simulink model "sixDOF4"  (R2024a)
settings: Solver=VariableStepAuto  StartTime=0.0  StopTime=30  MinStep=0.001  RelTol=1e-3
PreLoadFcn:
  | load("C:\Users\craig\OneDrive\Desktop\Matlab\TVC\Workspaces\rocketProps.mat");
values from neighbouring files (symbols this model uses):
  AoA = [-88.914 -74.145 -55.955 -43.246 -35.663 -31.356 -27.884 -25.044 -22.757 -21.029 -19.522 -18.257 ... (59 elements, 59x1)]    [rocketProps.mat]
  Cn = [-5.771 -4.929 -4.21 -3.639 -3.162 -2.748 -2.412 -2.115 -1.835 -1.564 -1.294 -1.003 ... (59 elements, 59x1)]    [rocketProps.mat]
  thrust = [13 82 98 100 90 86 93 96 96 92 88 83 ... (16 elements, 16x1)]    [rocketProps.mat]
  time = [0.01 0.02 0.03 0.04 0.05 0.06 0.12 0.2 0.3 0.7 0.9 1.07 ... (16 elements, 16x1)]    [rocketProps.mat]
undefined symbols (not defined in the file or in its folder): magnitude
libraries: sharedtransform x2, simulink x2, aerolibanim x1, vrlib x1
settings Model: NumberOfSteps=100  Creator=craig  LastModifiedBy=craig
settings SolverCC: MaxConsecutiveMinStep=2
settings DebuggingCC: UnderSpecifiedDataTypeMsg=warning  UnderSpecifiedDimensionMsg=warning

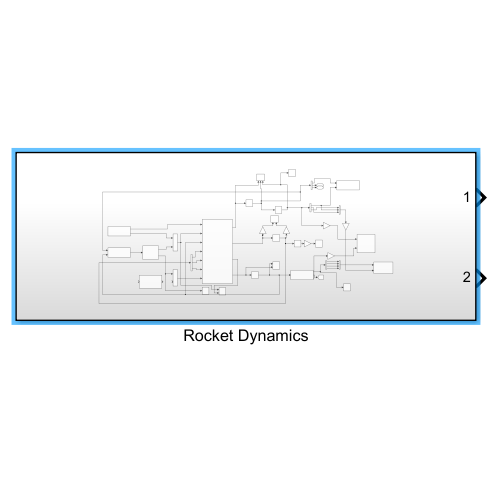
[thumbnail: Simulink's stored preview of the top-level diagram]
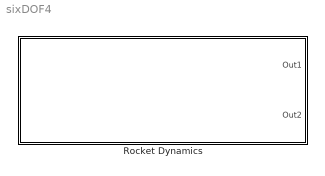
== system sixDOF4 ==
  Rocket Dynamics : Subsystem

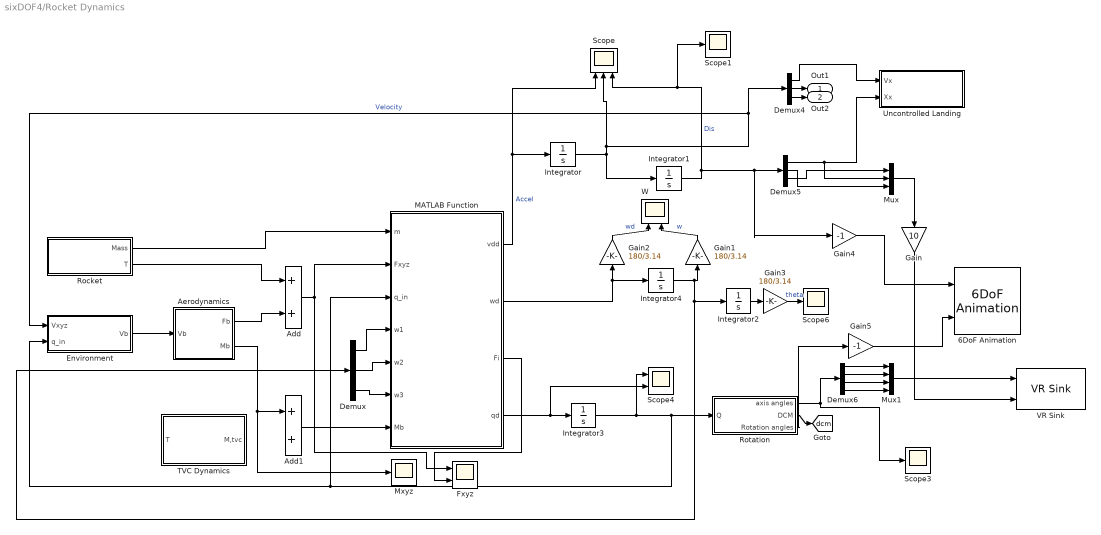
== system sixDOF4/Rocket Dynamics ==
  6DoF Animation : aerolibanim/6DoF Animation  u1=[0 4000 -2000 2000 -5000 -3000]  u2=0.1  u3=100  u4=[4000 0 -5000]  u5=Fixed position  u6=[2000 500 -3150]  u7=10  u8=on
  Add : Sum
  Add1 : Sum
  Aerodynamics : Subsystem
  Demux : Demux  Outputs=3
  Demux4 : Demux  Outputs=3
  Demux5 : Demux  Outputs=3
  Demux6 : Demux
  Environment : Subsystem
  Fxyz : Scope  NumInputPorts=2
  Gain : Gain  Gain=10
  Gain1 : Gain  Gain=180/3.14
  Gain2 : Gain  Gain=180/3.14
  Gain3 : Gain  Gain=180/3.14
  Gain4 : Gain  Gain=-1
  Gain5 : Gain  Gain=-1
  Integrator : Integrator  InitialCondition=[0; 0; 0]
  Integrator1 : Integrator
  Integrator2 : Integrator  InitialCondition=[0; 0; 0]
  Integrator3 : Integrator  InitialCondition=[1; 0; 0; 0]
  Integrator4 : Integrator  InitialCondition=[0; 0; 0]
  MATLAB Function : MATLAB Function  TreatAsAtomicUnit=on
  Mux : Mux  Inputs=3
  Mux1 : Mux
  Mxyz : Scope
  Rocket : Subsystem
  Rotation : Subsystem
  Scope : Scope  NumInputPorts=3
  Scope1 : Scope
  Scope3 : Scope
  Scope4 : Scope  NumInputPorts=2
  Scope6 : Scope
  TVC Dynamics : Subsystem
  Uncontrolled Landing : Subsystem
  VR Sink : vrlib/VR Sink  InstantiateOnLoad=on  SampleTime=0.1  ViewEnable=on  RemoteChange=off  RemoteView=off  FieldsWritten=MyTransform.rotation.4.1.1.double#MyTransform.translation.3.1.1.double  WorldFileName=C:\Users\craig\OneDrive\Desktop\Matlab\TVC\Animations\BestViewpoint.wrl  AutoView=off  VideoDimensions=[]  AllowVariableSize=off
  W : Scope  NumInputPorts=2
  Out1 : Outport
  Out2 : Outport  Port=2
  tag scope: dcm=global
  wires:
  Integrator3/1 -> Scope4/1, Rotation/1(Q), MATLAB Function/3(q_in), Environment/2(q_in)
  Add/1 -> Fxyz/1, MATLAB Function/2(Fxyz)
  Integrator2/1 -> Gain3/1
  Integrator4/1 -> Integrator2/1, Demux/1, Gain1/1
  Integrator/1 -> Integrator1/1, Demux4/1, Environment/1(Vxyz), Scope/2  "Velocity"
  Demux/1 -> MATLAB Function/4(w1)
  Integrator1/1 -> Scope1/1, Scope/3, Gain4/1, Demux5/1  "Dis"
  Demux5/1 -> Uncontrolled Landing/2(Xx), Mux/2
  MATLAB Function/3(Fi) -> Fxyz/2
  Environment/1("Vb ") -> Aerodynamics/1(Vb)
  Gain/1 -> VR Sink/2
  Mux/1 -> Gain/1
  Gain3/1 -> Scope6/1  "theta"
  Demux/3 -> MATLAB Function/6(w3)
  MATLAB Function/1(vdd) -> Integrator/1, Scope/1  "Accel"
  Aerodynamics/2(Mb) -> Add1/1, Mxyz/1
  Demux/2 -> MATLAB Function/5(w2)
  Demux4/3 -> Out2/1
  MATLAB Function/2(wd) -> Integrator4/1, Gain2/1
  MATLAB Function/4(qd) -> Scope4/2, Integrator3/1
  Rotation/1(axis angles) -> Scope3/1, Demux6/1
  Rocket/2(T) -> Add/1
  Gain1/1 -> W/2  "w"
  Rocket/1(Mass) -> MATLAB Function/1(m)
  Aerodynamics/1(Fb) -> Add/2
  Gain2/1 -> W/1  "wd"
  Rotation/2(DCM) -> [dcm]
  Demux4/1 -> Uncontrolled Landing/1(Vx)
  Rotation/3(Rotation angles) -> Gain5/1
  Gain4/1 -> 6DoF Animation/1
  Gain5/1 -> 6DoF Animation/2
  Demux4/2 -> Out1/1
  Add1/1 -> MATLAB Function/7(Mb)
  Mux1/1 -> VR Sink/1
  Demux5/3 -> Mux/1
  Demux5/2 -> Mux/3
  Demux6/2 -> Mux1/2
  Demux6/3 -> Mux1/3
  Demux6/1 -> Mux1/1
  Demux6/4 -> Mux1/4

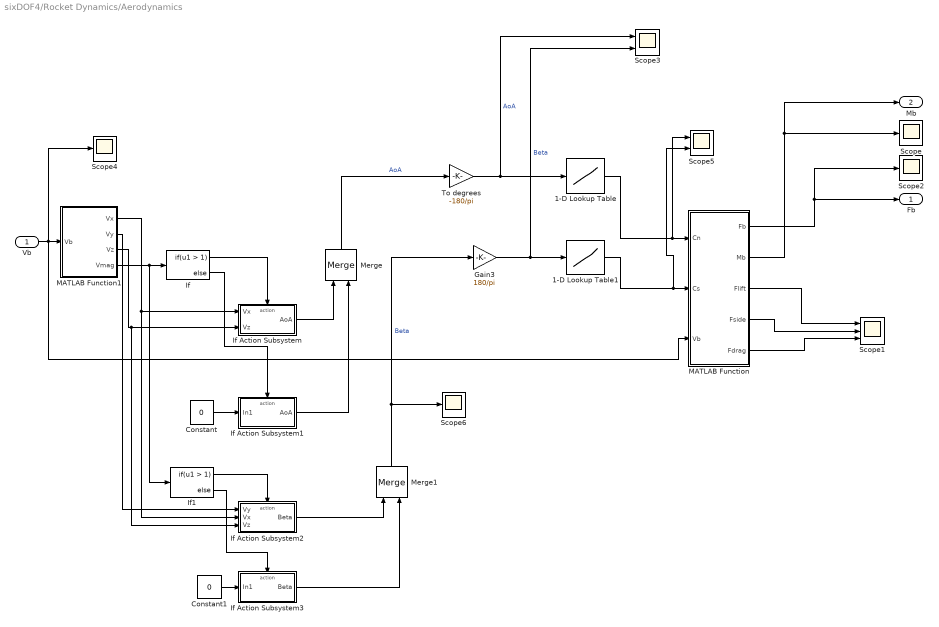
== system sixDOF4/Rocket Dynamics/Aerodynamics ==
  Vb : Inport
  1-D Lookup Table : Lookup_n-D  NumberOfTableDimensions=1  BreakpointsForDimension1=AoA  Table=Cn  InternalRulePriority=Speed  RndMeth=Simplest
  1-D Lookup Table1 : Lookup_n-D  NumberOfTableDimensions=1  BreakpointsForDimension1=AoA  Table=Cn  InternalRulePriority=Speed  RndMeth=Simplest
  Constant : Constant  Value=0
  Constant1 : Constant  Value=0
  Gain3 : Gain  Gain=180/pi
  If : If  IfExpression=u1 > 1
  If Action Subsystem : Subsystem  TreatAsAtomicUnit=on
  If Action Subsystem1 : Subsystem  TreatAsAtomicUnit=on
  If Action Subsystem2 : Subsystem  TreatAsAtomicUnit=on
  If Action Subsystem3 : Subsystem  TreatAsAtomicUnit=on
  If1 : If  IfExpression=u1 > 1
  MATLAB Function : MATLAB Function  TreatAsAtomicUnit=on
  MATLAB Function1 : MATLAB Function  TreatAsAtomicUnit=on
  Merge : Merge
  Merge1 : Merge
  Scope{,2,4,6} (4 alike) : Scope
  Scope1 : Scope  NumInputPorts=3
  Scope3 : Scope  NumInputPorts=2
  Scope5 : Scope  NumInputPorts=2
  To degrees : Gain  Gain=-180/pi
  Fb : Outport
  Mb : Outport  Port=2
  wires:
  MATLAB Function/3(Flift) -> Scope1/1
  MATLAB Function/2(Mb) -> Scope/1, Mb/1
  MATLAB Function/1(Fb) -> Scope2/1, Fb/1
  To degrees/1 -> Scope3/1, 1-D Lookup Table/1  "AoA"
  Gain3/1 -> Scope3/2, 1-D Lookup Table1/1  "Beta"
  MATLAB Function/5(Fdrag) -> Scope1/3
  Vb/1 -> Scope4/1, MATLAB Function/3(Vb), MATLAB Function1/1(Vb)
  If/2 -> If Action Subsystem1/Action
  MATLAB Function1/4(Vmag) -> If1/1, If/1
  Constant/1 -> If Action Subsystem1/1(In1)
  MATLAB Function1/1(Vx) -> If Action Subsystem2/2(Vx), If Action Subsystem/1(Vx)
  MATLAB Function1/3(Vz) -> If Action Subsystem2/3(Vz), If Action Subsystem/2(Vz)
  If/1 -> If Action Subsystem/Action
  If Action Subsystem/1(AoA) -> Merge/1
  If Action Subsystem1/1(AoA) -> Merge/2
  Merge/1 -> To degrees/1  "AoA"
  MATLAB Function1/2(Vy) -> If Action Subsystem2/1(Vy)
  Constant1/1 -> If Action Subsystem3/1(In1)
  If Action Subsystem2/1(Beta) -> Merge1/1
  If Action Subsystem3/1(Beta) -> Merge1/2
  If1/2 -> If Action Subsystem3/Action
  If1/1 -> If Action Subsystem2/Action
  1-D Lookup Table1/1 -> Scope5/2, MATLAB Function/2(Cs)
  1-D Lookup Table/1 -> Scope5/1, MATLAB Function/1(Cn)
  MATLAB Function/4(Fside) -> Scope1/2
  Merge1/1 -> Gain3/1, Scope6/1  "Beta"

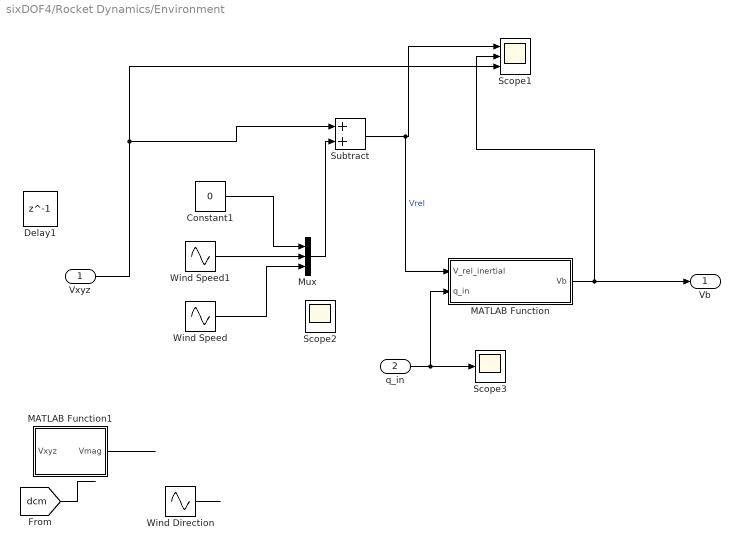
== system sixDOF4/Rocket Dynamics/Environment ==
  Vxyz : Inport
  q_in : Inport  Port=2
  Constant1 : Constant  Value=0
  Delay1 : Delay  DelayLength=1
  MATLAB Function : MATLAB Function  TreatAsAtomicUnit=on
  MATLAB Function1 : MATLAB Function  TreatAsAtomicUnit=on
  Mux : Mux  Inputs=3
  Scope1 : Scope  NumInputPorts=3
  Scope2 : Scope
  Scope3 : Scope
  Subtract : Sum
  Wind Direction : Sin  Amplitude=5  Bias=45  Frequency=2*pi*0.25  SampleTime=0
  Wind Speed : Sin  Amplitude=5  Bias=3.5  Frequency=2*pi*0.25  SampleTime=0
  Wind Speed1 : Sin  Amplitude=5  Bias=3.5  Frequency=2*pi*0.25  SampleTime=0
  "Vb " : Outport
  wires:
  Subtract/1 -> MATLAB Function/1(V_rel_inertial), Scope1/1  "Vrel"
  Vxyz/1 -> Subtract/1, Scope1/3
  [dcm] -> ?
  MATLAB Function1/1(Vmag) -> ?
  MATLAB Function/1(Vb) -> "Vb "/1, Scope1/2
  Wind Direction/1 -> ?
  Constant1/1 -> Mux/1
  q_in/1 -> MATLAB Function/2(q_in), Scope3/1
  Mux/1 -> Subtract/2
  Wind Speed1/1 -> Mux/2
  Wind Speed/1 -> Mux/3

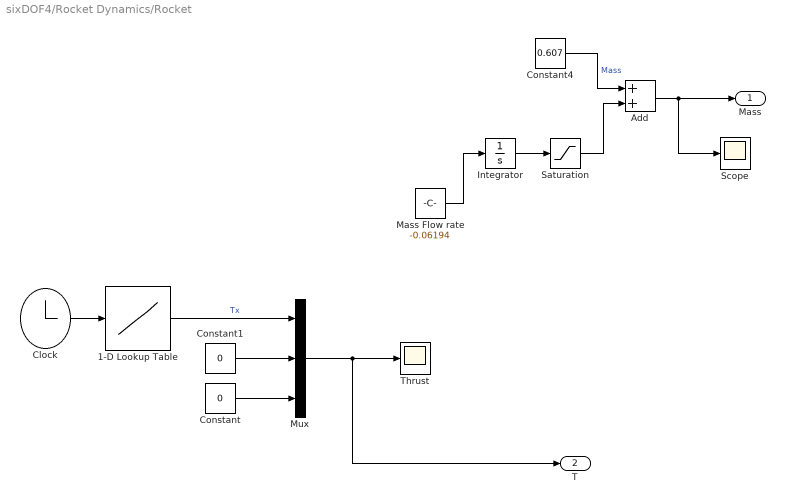
== system sixDOF4/Rocket Dynamics/Rocket ==
  1-D Lookup Table : Lookup_n-D  NumberOfTableDimensions=1  BreakpointsForDimension1=time  Table=thrust  TableMin=[0]  TableDataTypeStr=Inherit: Inherit from 'Table data'  ExtrapMethod=Clip  UseLastTableValue=on  InternalRulePriority=Speed  RndMeth=Simplest
  Add : Sum
  Clock : Clock
      settings: Decimation=100
  Constant : Constant  Value=0
  Constant1 : Constant  Value=0
  Constant4 : Constant  Value=0.607
  Integrator : Integrator  InitialCondition=0.188
  Mass Flow rate : Constant  Value=-0.06194
  Mux : Mux  Inputs=3
  Saturation : Saturate  LowerLimit=0.105
  Scope : Scope
  Thrust : Scope
  Mass : Outport
  T : Outport  Port=2
  wires:
  Clock/1 -> 1-D Lookup Table/1
  Constant1/1 -> Mux/2
  Mux/1 -> T/1, Thrust/1
  Constant4/1 -> Add/1  "Mass"
  Add/1 -> Scope/1, Mass/1
  1-D Lookup Table/1 -> Mux/1  "Tx"
  Constant/1 -> Mux/3
  Mass Flow rate/1 -> Integrator/1
  Integrator/1 -> Saturation/1
  Saturation/1 -> Add/2

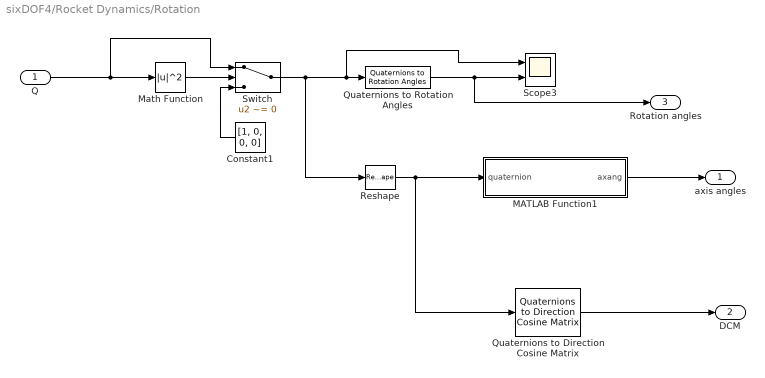
== system sixDOF4/Rocket Dynamics/Rotation ==
  Q : Inport
  Constant1 : Constant  Value=[1, 0, 0, 0]
  MATLAB Function1 : MATLAB Function  TreatAsAtomicUnit=on
  Math Function : Math  Operator=magnitude^2
  Quaternions to Direction Cosine Matrix : sharedtransform/Quaternions to  Direction Cosine Matrix  aMode=aMode
      settings: LibrarySourceBlock=|
      | aerolibtransform2/Quaternions to
      | Direction Cosine Matrix
  Quaternions to Rotation Angles : sharedtransform/Quaternions to Rotation Angles  rotationOrder=XYZ  aMode=aMode
  Reshape : Reshape  OutputDimensionality=Customize  OutputDimensions=[1,4]
  Scope3 : Scope  NumInputPorts=2
  Switch : Switch  Criteria=u2 ~= 0  SaturateOnIntegerOverflow=off  InputSameDT=off
  axis angles : Outport
  DCM : Outport  Port=2
  Rotation angles : Outport  Port=3
  wires:
  Constant1/1 -> Switch/3
  Quaternions to Rotation Angles/1 -> Rotation angles/1, Scope3/2
  Switch/1 -> Reshape/1, Scope3/1, Quaternions to Rotation Angles/1
  Math Function/1 -> Switch/2
  Q/1 -> Switch/1, Math Function/1
  MATLAB Function1/1(axang) -> axis angles/1
  Reshape/1 -> Quaternions to Direction Cosine Matrix/1, MATLAB Function1/1(quaternion)
  Quaternions to Direction Cosine Matrix/1 -> DCM/1

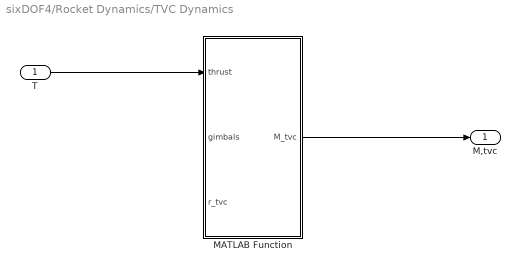
== system sixDOF4/Rocket Dynamics/TVC Dynamics ==
  T : Inport
  MATLAB Function : MATLAB Function  TreatAsAtomicUnit=on
  M,tvc : Outport
  wires:
  MATLAB Function/1(M_tvc) -> M,tvc/1
  T/1 -> MATLAB Function/1(thrust)

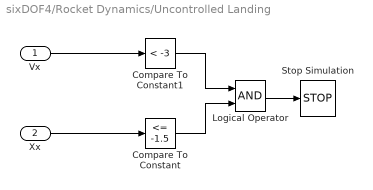
== system sixDOF4/Rocket Dynamics/Uncontrolled Landing ==
  Vx : Inport
  Xx : Inport  Port=2
  Compare To Constant : simulink/Logic and Bit Operations/Compare To Constant  relop=<=  const=-1.5  OutDataTypeStr=boolean
  Compare To Constant1 : simulink/Logic and Bit Operations/Compare To Constant  relop=<  const=-3  OutDataTypeStr=boolean
  Logical Operator : Logic  AllPortsSameDT=off  OutDataTypeStr=boolean
  Stop Simulation : Stop
  wires:
  Compare To Constant/1 -> Logical Operator/2
  Vx/1 -> Compare To Constant1/1
  Xx/1 -> Compare To Constant/1
  Compare To Constant1/1 -> Logical Operator/1
  Logical Operator/1 -> Stop Simulation/1

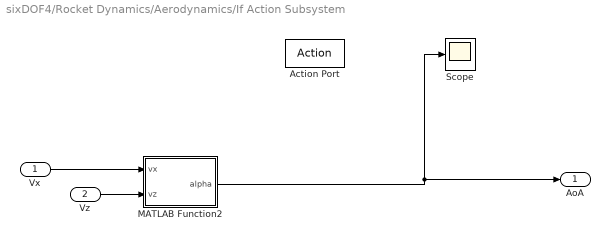
== system sixDOF4/Rocket Dynamics/Aerodynamics/If Action Subsystem ==
  Vx : Inport
  Vz : Inport  Port=2
  Action Port : ActionPort  ActionPortLabel=if(u1 > 1)
  MATLAB Function2 : MATLAB Function  TreatAsAtomicUnit=on
  Scope : Scope
  AoA : Outport
  wires:
  MATLAB Function2/1(alpha) -> Scope/1, AoA/1
  Vx/1 -> MATLAB Function2/1(vx)
  Vz/1 -> MATLAB Function2/2(vz)

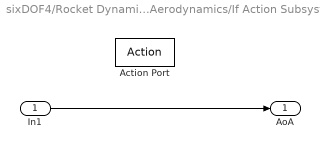
== system sixDOF4/Rocket Dynamics/Aerodynamics/If Action Subsystem1 ==
  In1 : Inport
  Action Port : ActionPort  ActionPortLabel=else
  AoA : Outport
  wires:
  In1/1 -> AoA/1

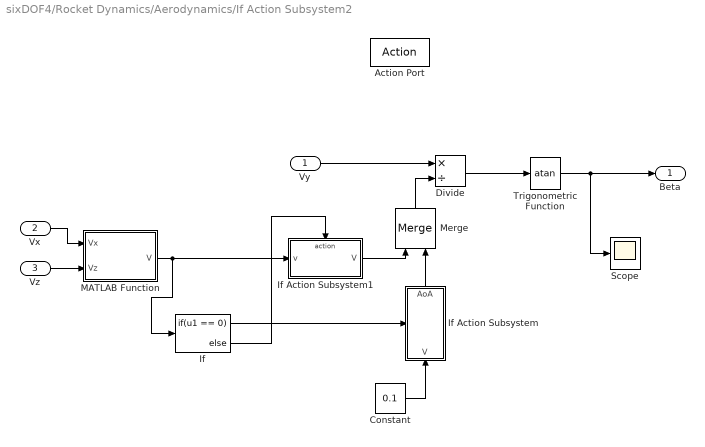
== system sixDOF4/Rocket Dynamics/Aerodynamics/If Action Subsystem2 ==
  Vy : Inport
  Vx : Inport  Port=2
  Vz : Inport  Port=3
  Action Port : ActionPort  ActionPortLabel=if(u1 > 1)
  Constant : Constant  Value=0.1
  Divide : Product  Inputs=*/
  If : If  IfExpression=u1 == 0
  If Action Subsystem : Subsystem  TreatAsAtomicUnit=on
  If Action Subsystem1 : Subsystem  TreatAsAtomicUnit=on
  MATLAB Function : MATLAB Function  TreatAsAtomicUnit=on
  Merge : Merge
  Scope : Scope
  Trigonometric Function : Trigonometry  Operator=atan
  Beta : Outport
  wires:
  Vx/1 -> MATLAB Function/1(Vx)
  Vz/1 -> MATLAB Function/2(Vz)
  Divide/1 -> Trigonometric Function/1
  Vy/1 -> Divide/1
  Constant/1 -> If Action Subsystem/1(V)
  Trigonometric Function/1 -> Scope/1, Beta/1
  If/1 -> If Action Subsystem/Action
  If Action Subsystem/1(AoA) -> Merge/2
  If/2 -> If Action Subsystem1/Action
  If Action Subsystem1/1(V) -> Merge/1
  Merge/1 -> Divide/2
  MATLAB Function/1(V) -> If/1, If Action Subsystem1/1(v)

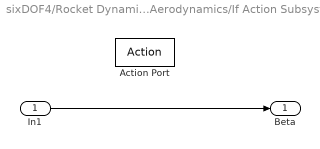
== system sixDOF4/Rocket Dynamics/Aerodynamics/If Action Subsystem3 ==
  In1 : Inport
  Action Port : ActionPort  ActionPortLabel=else
  Beta : Outport
  wires:
  In1/1 -> Beta/1

== system sixDOF4/Rocket Dynamics/Aerodynamics/If Action Subsystem2/If Action Subsystem ==
  V : Inport
  Action Port : ActionPort  ActionPortLabel=if(u1 == 0)
  AoA : Outport
  wires:
  V/1 -> AoA/1

== system sixDOF4/Rocket Dynamics/Aerodynamics/If Action Subsystem2/If Action Subsystem1 ==
  v : Inport
  Action Port : ActionPort  ActionPortLabel=else
  V : Outport
  wires:
  v/1 -> V/1

== matlab function sixDOF4/Rocket Dynamics/TVC Dynamics/MATLAB Function ==
  data: thrust input; M_tvc output; gimbals input; r_tvc input
function M_tvc = TVC_Controller(thrust, gimbals, r_tvc)


%TVC_Controller: Computes the thrust vector and the resulting moment

theta = 0; %gimbals(1);
psi = 0; %gimbals(2);

    % Define the thrust vector in the body frame
    %TVC_body = thrust * [cos(theta) * cos(psi);  sin(psi); sin(theta)];
    
    % Calculate the moment arm (r_tvc cross T_body)
    %M_tvc = cross(r_tvc, TVC_body);
    M_tvc = [0; 0; 0;];

end

== matlab function sixDOF4/Rocket Dynamics/Aerodynamics/If Action Subsystem/MATLAB Function2 ==
  data: vx input; alpha output; vz input
function alpha = fcn(vx, vz)

if norm(vx) < 0.1 && norm(vz) < 0.1
    alpha = 0;
else
    alpha = atan2(vz, vx);
end

== matlab function sixDOF4/Rocket Dynamics/MATLAB Function ==
  data: m input; Fxyz input; q_in input size=4; w1 input; w2 input; w3 input; Mb input; vdd output size=[3,1]; wd output size=[3,1]; Fi output; qd output
function [vdd, wd, Fi, qd] = EOM(m, Fxyz, q_in, w1, w2, w3, Mb)

q_in = q_in / norm(q_in);

Ix=0.00083;
Iy=0.10401;
Iz=0.10401;
g=9.81;
wx=w1;
wy=w2;
wz=w3;
w=[w1;w2;w3];

%Angular accelerations using newtons 2nd law for rotations in body frame
wxd = (1/Ix) * (Mb(1) + (Iy - Iz) * wy * wz);
wyd = (1/Iy) * (Mb(2) + (Iz - Ix) * wx * wz);
wzd = (1/Iz) * (Mb(3) + (Ix - Iy) * wx * wy);
wd =[wxd;wyd;wzd];


%update quaternion to reflect attitude change using formula for RoC of
%quaternion
qd=0.5*hamilton(q_in,[0;wx;wy;wz]);

% Net force from body to inertial frame (thrust + drag) accounting for change of
% attitude from drag

Fi_quat = hamilton(hamilton(q_in, [0; Fxyz]), conjugate(q_in));  % Reverse the order of quaternion transformation
Fi = Fi_quat(2:4); %remove scalar


% Translational accelerations
% Compute the translational accelerations, accounting for rotational coupling
xdd = (Fi(1) / m) - g;
ydd = Fi(2) / m;      
zdd = (Fi(3) / m);    

vdd = [xdd; ydd; zdd];


function product = hamilton(q, r)
    product = [r(1)*q(1) - r(2)*q(2) - r(3)*q(3) - r(4)*q(4);
               r(1)*q(2) + r(2)*q(1) + r(3)*q(4) - r(4)*q(3);
               r(1)*q(3) - r(2)*q(4) + r(3)*q(1) + r(4)*q(2);
               r(1)*q(4) + r(2)*q(3) - r(3)*q(2) + r(4)*q(1)];
end

%create a function to multiply quaternions  
 %   function product=hamilton(q,r)
   %     product=[r(1)*q(1)-r(2)*q(2)-r(3)*q(3)-r(4)*q(4);
   %              r(1)*q(2)+r(2)*q(1)-r(3)*q(4)+r(4)*q(3);
   %              r(1)*q(3)+r(2)*q(4)+r(3)*q(1)-r(4)*q(2);
  %               r(1)*q(4)-r(2)*q(3)+r(3)*q(2)+r(4)*q(1)];
   % end

%calculate conjugate of quaternion
    function q_star=conjugate(q)
        q_star=[q(1);-q(2);-q(3);-q(4)];
    end

end

== matlab function sixDOF4/Rocket Dynamics/Aerodynamics/MATLAB Function ==
  data: Fb output size=3; Mb output size=3; Cn input; Cs input; Flift output size=1; Fside output; Vb input size=3; Fdrag output size=3
function [Fb, Mb, Flift, Fside, Fdrag] = Lift(Cn, Cs, Vb)

Length = 1.25;
Ab = 0.003504635;
l = 0.202;
Mroll = 0;
rho = 1.225;
Cdx = 0.4;
Cdyz = 1.3;
d = 0.068;
Vbx = Vb(1);
Vby = Vb(2);
Vbz = Vb(3);


q = 0.5 * rho * norm(Vb)^2;
% Drag force vector, opposing the velocity vector
if norm(Vb) > 0
    Fdragmagx = q * Ab * Cdx; 
    Fdragmagyz = q * Ab * Cdyz;
    Fdragx = Fdragmagx * (Vbx / norm(Vb));
    Fdragyz = Fdragmagyz * ([Vby; Vbz] / norm(Vb));
    Fdrag = [Fdragx; Fdragyz];
    Flift = q * Ab * Cn; %based off AoA
    Fside = q * Ab * Cs;  %based of sideslip/beta

else
   Fdrag = [0; 0; 0]; % No drag force when velocity is zero
   Flift = 0;  % No lift force when velocity is zero
   Fside = 0;  % No side force when velocity is zer0
end

%moment coefficients

Cmp = ((Cn * l)/d); %based of aoa 
Cmy = ((Cs * l)/d); %based of sideslip/beta

Mpitch = q * Ab * d * Cmp; %based of aoa 
Myaw = q * Ab * d * Cmy; %based of sideslip/beta

Mb = [Mroll; -Mpitch; -Myaw];

Fb =[0; -Fside; Flift] - Fdrag;

end

%rotation damping C's
%Cmpd = (-2 * Cn * l/Length); %another eq uses mach number to estimate
%Cmyd = (-2 * Cs * l/Length);
%Cmpd = -1/8 * d^2/Ab * m^2 / (1 + m^2);
%Cmyd = -1/8 * d^2/Ab * m^2 / (1 + m^2);
%C's for roc of AoA and beta angle
%CrAoAd = -(2 * CnAoA)/(pi* ARf);
%Cmybeta = (CnAoA)/(ARf);

%+ (d /(2*norm(Vb))) *(Cmpd)*w2; %+ CrAoAd removed
    %Cmy = -((Cs * l) / d ) + (d /(2*norm(Vb)))*(Cmyd + Cmybeta)*w3;

== matlab function sixDOF4/Rocket Dynamics/Environment/MATLAB Function ==
  data: V_rel_inertial input; Vb output; q_in input size=4
function Vb = I_to_b(V_rel_inertial, q_in)

q_in = q_in / norm(q_in);

% Transform velocity to body frame quaternion using current orientation
Vb_quat = hamilton(hamilton(conjugate(q_in), [0; V_rel_inertial]), q_in);
Vb = Vb_quat(2:4);  % Remove scalar part



%calculate conjugate of quaternion
    function q_star=conjugate(q)
        q_star=[q(1);-q(2);-q(3);-q(4)];
    end

end

function product = hamilton(q, r)
    product = [r(1)*q(1) - r(2)*q(2) - r(3)*q(3) - r(4)*q(4);
               r(1)*q(2) + r(2)*q(1) + r(3)*q(4) - r(4)*q(3);
               r(1)*q(3) - r(2)*q(4) + r(3)*q(1) + r(4)*q(2);
               r(1)*q(4) + r(2)*q(3) - r(3)*q(2) + r(4)*q(1)];
end

%create a function to multiply quaternions  
 %   function product=hamilton(q,r)
   %     product=[r(1)*q(1)-r(2)*q(2)-r(3)*q(3)-r(4)*q(4);
   %              r(1)*q(2)+r(2)*q(1)-r(3)*q(4)+r(4)*q(3);
   %              r(1)*q(3)+r(2)*q(4)+r(3)*q(1)-r(4)*q(2);
  %               r(1)*q(4)-r(2)*q(3)+r(3)*q(2)+r(4)*q(1)];
   % end

== matlab function sixDOF4/Rocket Dynamics/Rotation/MATLAB Function1 ==
  data: quaternion input; axang output
function axang = fcn(quaternion)
    rotm = quat2rotm(quaternion);
   
    
%As rotm2axang outputs a 4 element vector including axis/angle together
    axang = -rotm2axang(rotm);
    
end

== matlab function sixDOF4/Rocket Dynamics/Environment/MATLAB Function1 ==
  data: Vxyz input; Vmag output
function Vmag = mag(Vxyz)

Vmag = norm(Vxyz);

end

== matlab function sixDOF4/Rocket Dynamics/Aerodynamics/MATLAB Function1 ==
  data: Vx output; Vy output; Vz output; Vb input; Vmag output
function [Vx, Vy, Vz, Vmag]= mag(Vb)

Vx = Vb(1);
Vy = Vb(2);
Vz = Vb(3);

Vmag = norm(Vb);

end

== matlab function sixDOF4/Rocket Dynamics/Aerodynamics/If Action Subsystem2/MATLAB Function ==
  data: Vx input; V output; Vz input
function V = fcn(Vx, Vz)

Vyz = [Vx; Vz];
V = norm(Vyz);
